simulink model "Shuttle_Valve"  (R2016a)
settings: Solver=VariableStepAuto  SolverMode=SingleTasking  StartTime=0.0  StopTime=10.0  RelTol=1e-3
libraries: simulink x2
settings Model: Creator=James  LastModifiedBy=James
settings DebuggingCC: SFUnexpectedBacktrackingDiag=error  SFNoUnconditionalDefaultTransitionDiag=error
settings GRTTargetCC: TargetLangStandard=C99 (ISO)  GeneratePreprocessorConditionals=Use local settings
settings ConfigComp: CovMetricSettings=dwe  CovHtmlReporting=off  CovSaveCumulativeToWorkspaceVar=off  CovSaveSingleToWorkspaceVar=off  CovExternalEMLEnable=on

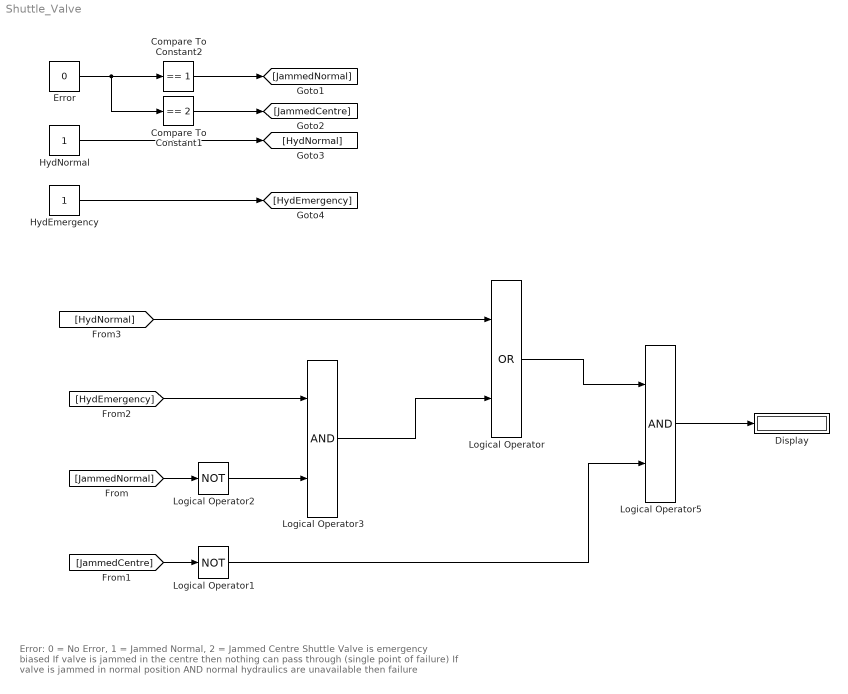
== system Shuttle_Valve ==
  note: Error: 0 = No Error, 1 = Jammed Normal, 2 = Jammed Centre
      |
      | Shuttle Valve is emergency biased
      |
      | If valve is jammed in the centre then nothing can pass through (single point of failure)
      |
      | If valve is jammed in normal position AND normal hydraulics are unavailable then failure
  Compare To Constant1 : simulink/Logic and Bit Operations/Compare To Constant  relop===  const=2  OutDataTypeStr=boolean
  Compare To Constant2 : simulink/Logic and Bit Operations/Compare To Constant  relop===  const=1  OutDataTypeStr=boolean
  Display : Display
  Error : Constant  Value=0  OutDataTypeStr=double
  HydEmergency : Constant  OutDataTypeStr=boolean
  HydNormal : Constant  OutDataTypeStr=double
  Logical Operator : Logic  Operator=OR  AllPortsSameDT=off  OutDataTypeStr=boolean
  Logical Operator1 : Logic  Operator=NOT  AllPortsSameDT=off  OutDataTypeStr=boolean
  Logical Operator2 : Logic  Operator=NOT  AllPortsSameDT=off  OutDataTypeStr=boolean
  Logical Operator3 : Logic  AllPortsSameDT=off  OutDataTypeStr=boolean
  Logical Operator5 : Logic  AllPortsSameDT=off  OutDataTypeStr=boolean
  wires:
  Error/1 -> Compare To Constant1/1, Compare To Constant2/1
  Compare To Constant2/1 -> [JammedNormal]
  Compare To Constant1/1 -> [JammedCentre]
  [JammedNormal] -> Logical Operator2/1
  Logical Operator2/1 -> Logical Operator3/2
  Logical Operator3/1 -> Logical Operator/2
  [JammedCentre] -> Logical Operator1/1
  Logical Operator/1 -> Logical Operator5/1
  Logical Operator1/1 -> Logical Operator5/2
  Logical Operator5/1 -> Display/1
  [HydEmergency] -> Logical Operator3/1
  HydNormal/1 -> [HydNormal]
  HydEmergency/1 -> [HydEmergency]
  [HydNormal] -> Logical Operator/1
